simulink model "control_temperatura"  (R2021a)
settings: Solver=VariableStepAuto  StartTime=0.0  StopTime=1000  RelTol=1e-3
libraries: fuzblock x1
settings Model: Creator=Bremdows  LastModifiedBy=Bremdows
settings OptimizationCC: BlockReduction=off  DefaultParameterBehavior=Inlined  BufferReuse=off

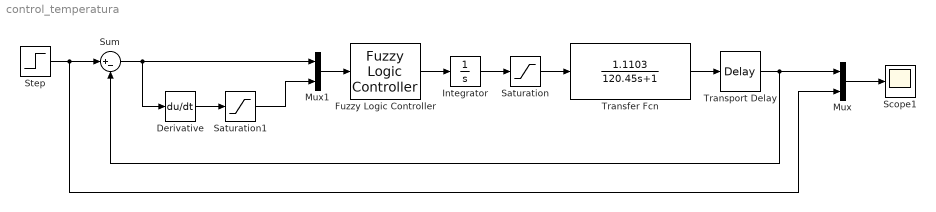
== system control_temperatura ==
  Derivative : Derivative
  Fuzzy Logic Controller : fuzblock/Fuzzy Logic  Controller  FIS='fuzzy_temperatura.fis'  OutputSampleNumber=101  DataType=double  FuzzifiedInputs=off  RuleFiringStrengths=off  RuleOutputs=off  AggregatedOutputs=off  SimulateUsing=Interpreted execution  OutOfRangeInputValueMessage=warning  NoRuleFiredMessage=warning  EmptyOutputFuzzySetMessage=warning
  Integrator : Integrator
  Mux : Mux  Inputs=2
  Mux1 : Mux  Inputs=2
  Saturation : Saturate
  Saturation1 : Saturate
  Scope1 : Scope
  Step : Step  Time=0  After=0.1  SampleTime=0
  Sum : Sum  Inputs=|+-
  Transfer Fcn : TransferFcn  Numerator=[1.1103]  Denominator=[120.45 1]
  Transport Delay : TransportDelay  DelayTime=12.78
  wires:
  Mux/1 -> Scope1/1
  Step/1 -> Mux/2, Sum/1
  Transfer Fcn/1 -> Transport Delay/1
  Transport Delay/1 -> Sum/2, Mux/1
  Fuzzy Logic Controller/1 -> Integrator/1
  Integrator/1 -> Saturation/1
  Saturation/1 -> Transfer Fcn/1
  Mux1/1 -> Fuzzy Logic Controller/1
  Sum/1 -> Derivative/1, Mux1/1
  Derivative/1 -> Saturation1/1
  Saturation1/1 -> Mux1/2
